simulink model "generate_audio"  (Simulink 6.6)
settings: Solver=ode45  StartTime=0.0  StopTime=0.02  RelTol=1e-3
PreLoadFcn:
  | Fs = 48000;
  | code_init = [0 0 0 0 0 1 0 1 1 1];
StopFcn:
  | figure(1)
  | plot(signal);
  | xlabel('Samples');
  | ylabel('Amplitude');
  | legend('Signal');
  | axis([0 length(signal) -1.2 1.2]);
libraries: xbsIndex_r4 x32, dspwin32 x1
settings Model: Creator=lcrockett  LastModifiedBy=lcrockett

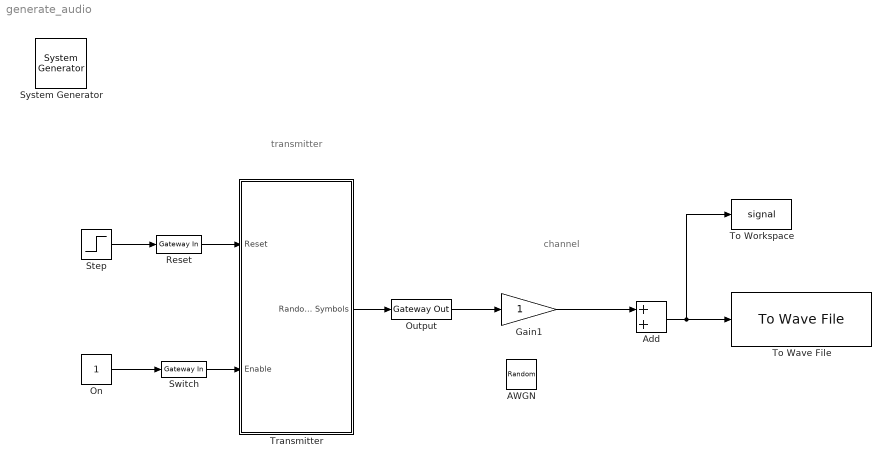
== system generate_audio ==
  note: channel
  note: transmitter
  " System Generator" : xbsIndex_r4/ System Generator  Tag=genX  SystemSampleTime=-1  xilinxfamily=virtex4  part=xc4vsx35  speed=-12  package=ff668  synthesis_tool=XST  clock_wrapper=Clock Enables  directory=./transmitter  testbench=off  simulink_period=1/Fs  sysclk_period=20  dcm_input_clock_period=100  incr_netlist=off  trim_vbits=Everywhere in SubSystem  dbl_ovrd=According to Block Masks  core_generation=According to Block Masks  run_coregen=off  deprecated_control=off  eval_field=0  block_type=sysgen
      settings: block_version=9.2.01
  AWGN : RandomNumber  Variance=0.1  Seed=56345  SampleTime=1/Fs
  Add : Sum  OutScaling=2^-10
  Gain1 : Gain
  On : Constant  SampleTime=21/Fs
  Output : xbsIndex_r4/Gateway Out  hdl_port=on  timing_constraint=None  locs_specified=off  LOCs={}  block_type=gatewayout
      settings: infoedit="Gateway out block.  Converts Xilinx fixed point inputs into ouputs of type Simulink integer, double, or fixed point.<P><P>Hardware notes:  In hardware these blocks become top level output ports or are discarded, depending on how they are configured."  block_version=8.2.02
  Reset : xbsIndex_r4/Gateway In  arith_type=Boolean  n_bits=16  bin_pt=14  quantization="Round  (unbiased: +/- Inf)"  overflow=Saturate  period=21/Fs  dbl_ovrd=off  timing_constraint=None  locs_specified=off  LOCs={}  block_type=gatewayin
      settings: infoedit="Gateway in block.  Converts inputs of type Simulink integer, double and fixed point to  Xilinx fixed point type.<P><P>Hardware notes:  In hardware these blocks become top level input ports."  block_version=8.2.02
  Step : Step  Time=10/Fs  Before=1  After=0  SampleTime=21/Fs
  Switch : xbsIndex_r4/Gateway In  arith_type=Boolean  n_bits=16  bin_pt=14  quantization="Round  (unbiased: +/- Inf)"  overflow=Saturate  period=21/Fs  dbl_ovrd=off  timing_constraint=None  locs_specified=off  LOCs={}  block_type=gatewayin
      settings: infoedit="Gateway in block.  Converts inputs of type Simulink integer, double and fixed point to  Xilinx fixed point type.<P><P>Hardware notes:  In hardware these blocks become top level input ports."  block_version=8.2.02
  To Wave File : dspwin32/To Wave File  filename=baseband_audio  sampleWidth=16  MinNumSamples=256
  To Workspace : ToWorkspace  VariableName=signal  SampleTime=-1  SaveFormat=Array
  Transmitter : Subsystem
  wires:
  Output/1 -> Gain1/1
  Step/1 -> Reset/1
  On/1 -> Switch/1
  Reset/1 -> Transmitter/1(Reset)
  Switch/1 -> Transmitter/2(Enable)
  Transmitter/1(Random Symbols) -> Output/1
  Gain1/1 -> Add/1
  Add/1 -> To Workspace/1, To Wave File/1

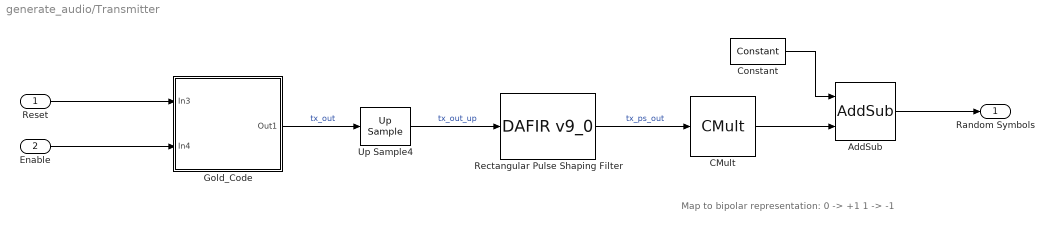
== system generate_audio/Transmitter ==
  note: Map to bipolar representation:
      | 0 -> +1
      | 1 -> -1
  Reset : Inport
  Enable : Inport  Port=2
  AddSub : xbsIndex_r4/AddSub  mode=Addition  use_carryin=off  use_carryout=off  en=off  latency=0  precision=Full  arith_type=Unsigned  n_bits=16  bin_pt=14  quantization=Truncate  overflow=Wrap  dbl_ovrd=off  use_behavioral_HDL=off  pipelined=off  use_rpm=on  block_type=addsub
      settings: block_version=10.1.2
  CMult : xbsIndex_r4/CMult  const=-2  const_n_bits=3  const_bin_pt=0  en=off  latency=0  precision=User Defined  arith_type="Signed  (2's comp)"  n_bits=3  bin_pt=0  quantization=Truncate  overflow=Wrap  dbl_ovrd=off  use_behavioral_HDL=off  mem_type=Distributed RAM  placement_style=Rectangular Shape  pipeline=off  use_rpm=off  block_type=cmult
      settings: block_version=10.1.2
  Constant : xbsIndex_r4/Constant  arith_type=Signed (2's comp)  const=1  n_bits=2  bin_pt=0  explicit_period=off  period=1  equ=P=C  opselect=C  inp2=PCIN>>17  opr=+  inp1=P  carry=CIN  dbl_ovrd=off  block_type=constant
      settings: block_version=10.1.2
  Gold_Code : Subsystem
  Rectangular Pulse Shaping Filter : xbsIndex_r4/DAFIR v9_0   coef=ones(1,21)  structure=Inferred from Coefficients  coef_n_bits=2  coef_bin_pt=0  over_sample=1  reload=off  valids=off  rst=off  latency=12  num_channels=1  serial_input=off  polyphase_behavior="Single Rate:  sample in - sample out"  dbl_ovrd=off  explicit_period=off  period=1  use_isim=0  block_type=fir
      settings: infoedit="Hardware notes: Implemented using distributed arithmetic (DA).  The hardware over sampling rate determines the degree of parallelism.  A rate of one produces a fully parallel DA filter.  A rate of n (resp., n+1) for an n-bit input signal produces a fully serial implementation for a non-symmetric (resp., symmetric) impulse response.  Intermediate values produce implementations with intermediate levels of parallelism."  block_version=9.1.01
  Up Sample4 : xbsIndex_r4/Up Sample  sample_ratio=21  copy_samples=off  dbl_ovrd=off  block_type=usamp
      settings: infoedit="Up samples input data.  Inserted values  can be zeros or copies of the most recent input sample.<P><P>Hardware notes: No hardware is needed if inserted values are copies of the input sample; otherwise, a mux and single bit flip-flop are used."  block_version=9.1.01
  Random Symbols : Outport
  wires:
  Up Sample4/1 -> Rectangular Pulse Shaping Filter/1  "tx_out_up"
  Reset/1 -> Gold_Code/1(In3)
  Rectangular Pulse Shaping Filter/1 -> CMult/1  "tx_ps_out"
  Enable/1 -> Gold_Code/2(In4)
  Gold_Code/1(Out1) -> Up Sample4/1  "tx_out"
  CMult/1 -> AddSub/2
  AddSub/1 -> Random Symbols/1
  Constant/1 -> AddSub/1

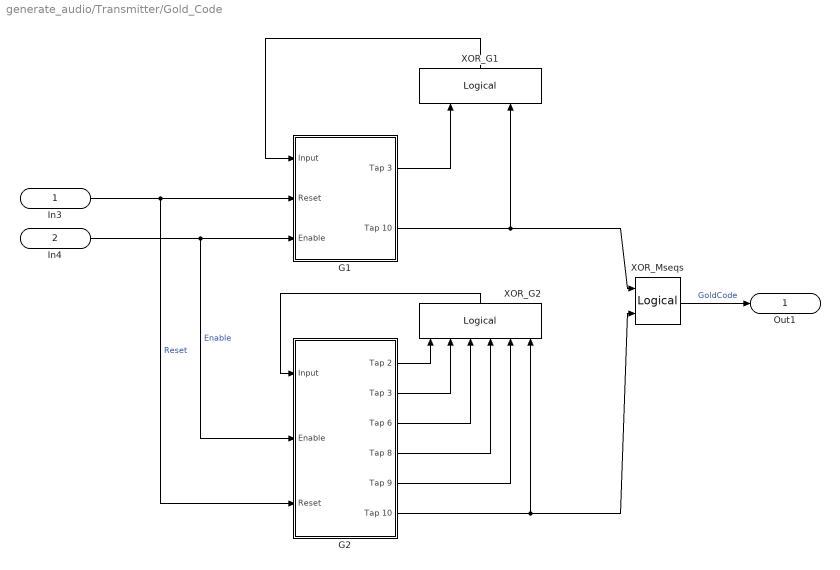
== system generate_audio/Transmitter/Gold_Code ==
  In3 : Inport
  In4 : Inport  Port=2
  G1 : Subsystem
  G2 : Subsystem
  XOR_G1 : xbsIndex_r4/Logical  Orientation=up  logical_function=XOR  inputs=2  en=off  latency=0  precision=User Defined  arith_type=Unsigned  n_bits=1  bin_pt=0  align_bp=on  dbl_ovrd=off  block_type=logical
      settings: block_version=8.2.01
  XOR_G2 : xbsIndex_r4/Logical  Orientation=up  logical_function=XOR  inputs=6  en=off  latency=0  precision=User Defined  arith_type=Unsigned  n_bits=1  bin_pt=0  align_bp=on  dbl_ovrd=off  block_type=logical
      settings: block_version=8.2.01
  XOR_Mseqs : xbsIndex_r4/Logical  logical_function=XOR  inputs=2  en=off  latency=0  precision=User Defined  arith_type=Unsigned  n_bits=1  bin_pt=0  align_bp=on  dbl_ovrd=off  block_type=logical
      settings: block_version=8.2.01
  Out1 : Outport
  wires:
  G1/1(Tap 3) -> XOR_G1/1
  XOR_G1/1 -> G1/1(Input)
  In3/1 -> G1/2(Reset), G2/3(Reset)  "Reset"
  XOR_Mseqs/1 -> Out1/1  "GoldCode"
  In4/1 -> G1/3(Enable), G2/2(Enable)  "Enable"
  G1/2(Tap 10) -> XOR_Mseqs/1, XOR_G1/2
  XOR_G2/1 -> G2/1(Input)
  G2/6(Tap 10) -> XOR_Mseqs/2, XOR_G2/6
  G2/1(Tap 2) -> XOR_G2/1
  G2/2(Tap 3) -> XOR_G2/2
  G2/3(Tap 6) -> XOR_G2/3
  G2/4(Tap 8) -> XOR_G2/4
  G2/5(Tap 9) -> XOR_G2/5

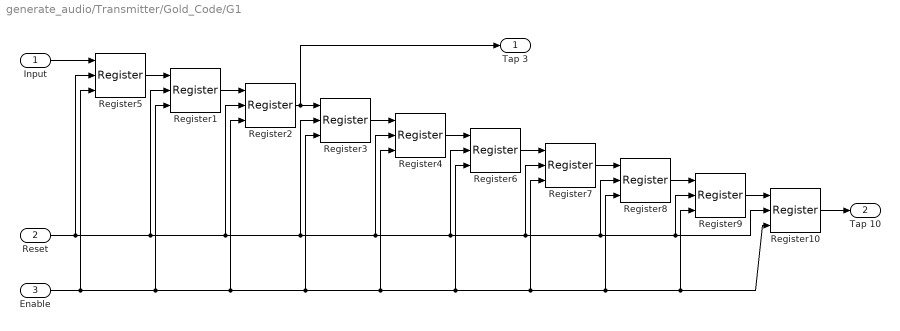
== system generate_audio/Transmitter/Gold_Code/G1 ==
  Input : Inport
  Reset : Inport  Port=2
  Enable : Inport  Port=3
  Register{1..10} (10 alike) : xbsIndex_r4/Register  init=1  rst=on  en=on  dbl_ovrd=off  block_type=register
      settings: block_version=8.2.01
  Tap 3 : Outport
  Tap 10 : Outport  Port=2
  wires:
  Reset/1 -> Register2/2, Register3/2, Register4/2, Register6/2, Register7/2, Register8/2, Register9/2, Register10/2, Register1/2, Register5/2
  Input/1 -> Register5/1
  Register3/1 -> Register4/1
  Register2/1 -> Register3/1, Tap 3/1
  Register1/1 -> Register2/1
  Register5/1 -> Register1/1
  Enable/1 -> Register1/3, Register3/3, Register4/3, Register6/3, Register7/3, Register8/3, Register9/3, Register10/3, Register2/3, Register5/3
  Register4/1 -> Register6/1
  Register6/1 -> Register7/1
  Register7/1 -> Register8/1
  Register8/1 -> Register9/1
  Register9/1 -> Register10/1
  Register10/1 -> Tap 10/1

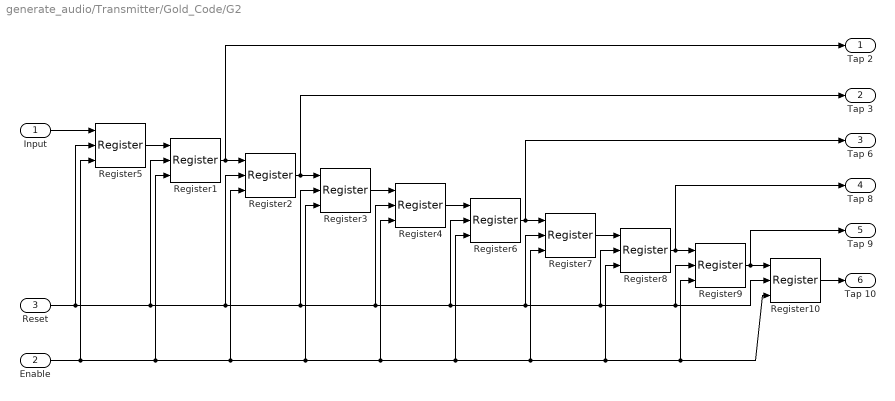
== system generate_audio/Transmitter/Gold_Code/G2 ==
  Input : Inport
  Enable : Inport  Port=2
  Reset : Inport  Port=3
  Register1 : xbsIndex_r4/Register  init=code_init(2)  rst=on  en=on  dbl_ovrd=off  block_type=register
      settings: block_version=8.2.01
  Register10 : xbsIndex_r4/Register  init=code_init(10)  rst=on  en=on  dbl_ovrd=off  block_type=register
      settings: block_version=8.2.01
  Register2 : xbsIndex_r4/Register  init=code_init(3)  rst=on  en=on  dbl_ovrd=off  block_type=register
      settings: block_version=8.2.01
  Register3 : xbsIndex_r4/Register  init=code_init(4)  rst=on  en=on  dbl_ovrd=off  block_type=register
      settings: block_version=8.2.01
  Register4 : xbsIndex_r4/Register  init=code_init(5)  rst=on  en=on  dbl_ovrd=off  block_type=register
      settings: block_version=8.2.01
  Register5 : xbsIndex_r4/Register  init=code_init(1)  rst=on  en=on  dbl_ovrd=off  block_type=register
      settings: block_version=8.2.01
  Register6 : xbsIndex_r4/Register  init=code_init(6)  rst=on  en=on  dbl_ovrd=off  block_type=register
      settings: block_version=8.2.01
  Register7 : xbsIndex_r4/Register  init=code_init(7)  rst=on  en=on  dbl_ovrd=off  block_type=register
      settings: block_version=8.2.01
  Register8 : xbsIndex_r4/Register  init=code_init(8)  rst=on  en=on  dbl_ovrd=off  block_type=register
      settings: block_version=8.2.01
  Register9 : xbsIndex_r4/Register  init=code_init(9)  rst=on  en=on  dbl_ovrd=off  block_type=register
      settings: block_version=8.2.01
  Tap 2 : Outport
  Tap 3 : Outport  Port=2
  Tap 6 : Outport  Port=3
  Tap 8 : Outport  Port=4
  Tap 9 : Outport  Port=5
  Tap 10 : Outport  Port=6
  wires:
  Reset/1 -> Register2/2, Register3/2, Register4/2, Register6/2, Register7/2, Register8/2, Register9/2, Register10/2, Register1/2, Register5/2
  Input/1 -> Register5/1
  Register3/1 -> Register4/1
  Register2/1 -> Register3/1, Tap 3/1
  Register1/1 -> Register2/1, Tap 2/1
  Register5/1 -> Register1/1
  Enable/1 -> Register1/3, Register3/3, Register4/3, Register6/3, Register7/3, Register8/3, Register9/3, Register10/3, Register2/3, Register5/3
  Register4/1 -> Register6/1
  Register6/1 -> Register7/1, Tap 6/1
  Register7/1 -> Register8/1
  Register8/1 -> Register9/1, Tap 8/1
  Register9/1 -> Register10/1, Tap 9/1
  Register10/1 -> Tap 10/1
